simulink model "Simulation_Nonlinear_MRAC"  (R2023b)
settings: Solver=VariableStepAuto  StartTime=0.0  StopTime=Tsim  RelTol=1e-3
undefined symbols (not defined in the file): a, am, amplitude, b, BETA, BETA_m, bias, bm, epsilon, frequency, IC_P, IC_Pm, period, phase_delay, pulse_width, SAT_ACTIVE, SIGNAL_NR, Tsim, w, WEIGHT_UPDATE, wm
libraries: simulink x1
settings Model: Creator=dalimwahby  LastModifiedBy=dalimwahby

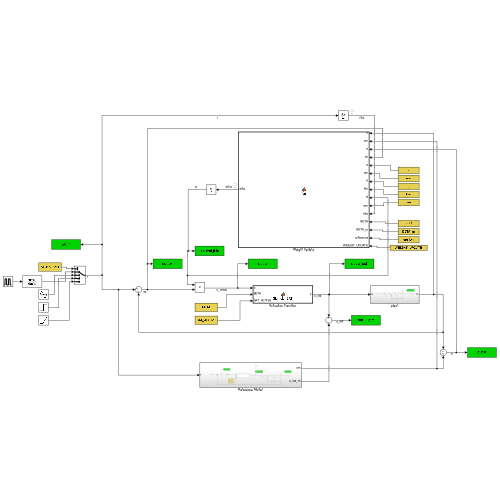
[thumbnail: Simulink's stored preview of the top-level diagram]
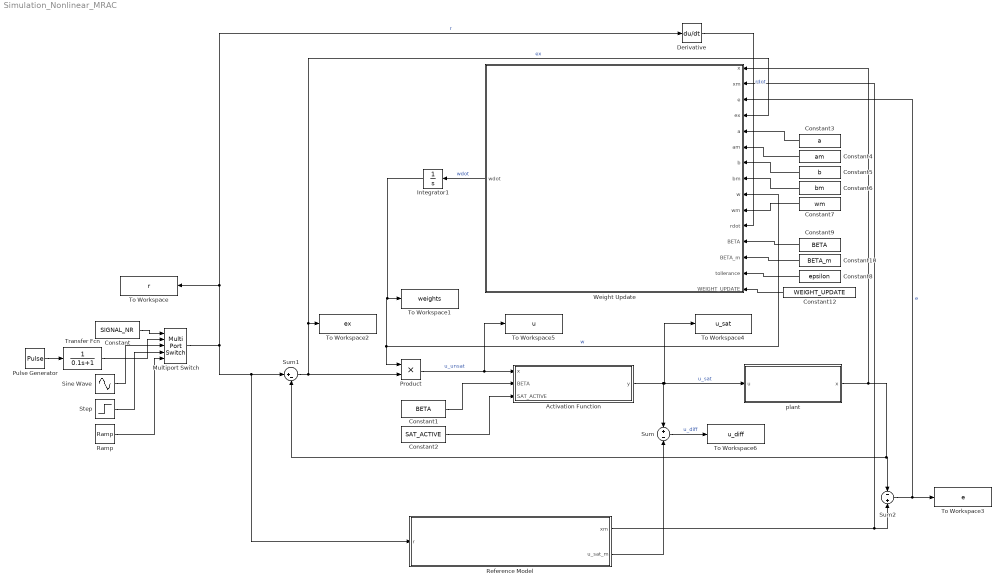
== system Simulation_Nonlinear_MRAC ==
  Activation Function : MATLAB Function  TreatAsAtomicUnit=on
  Constant : Constant  Value=SIGNAL_NR
  Constant1 : Constant  Value=BETA
  Constant10 : Constant  Value=BETA_m
  Constant12 : Constant  Value=WEIGHT_UPDATE
  Constant2 : Constant  Value=SAT_ACTIVE
  Constant3 : Constant  Value=a
  Constant4 : Constant  Value=am
  Constant5 : Constant  Value=b
  Constant6 : Constant  Value=bm
  Constant7 : Constant  Value=wm
  Constant8 : Constant  Value=epsilon
  Constant9 : Constant  Value=BETA
  Derivative : Derivative
  Integrator1 : Integrator  InitialCondition=w
  Multiport Switch : MultiPortSwitch  Inputs=4  SaturateOnIntegerOverflow=off  InputSameDT=off
  Product : Product
  Pulse Generator : DiscretePulseGenerator  PulseType=Time based  Amplitude=amplitude  Period=period  PulseWidth=pulse_width*100  PhaseDelay=phase_delay
  Ramp : simulink/Sources/Ramp  slope=1/Tsim  start=0  InitialOutput=0
  Reference Model : Subsystem
  Sine Wave : Sin  Amplitude=amplitude  Bias=bias  Frequency=frequency  SampleTime=0
  Step : Step  Time=phase_delay  After=amplitude  SampleTime=0
  Sum : Sum  Inputs=+-
  Sum1 : Sum  Inputs=|+-
  Sum2 : Sum  Inputs=-+
  To Workspace : ToWorkspace  VariableName=r  SaveFormat=Timeseries  SampleTime=-1
  To Workspace1 : ToWorkspace  VariableName=weights  SaveFormat=Timeseries  SampleTime=-1
  To Workspace2 : ToWorkspace  VariableName=ex  SaveFormat=Timeseries  SampleTime=-1
  To Workspace3 : ToWorkspace  VariableName=e  SaveFormat=Timeseries  SampleTime=-1
  To Workspace4 : ToWorkspace  VariableName=u_sat  SaveFormat=Timeseries  SampleTime=-1
  To Workspace5 : ToWorkspace  VariableName=u  SaveFormat=Timeseries  SampleTime=-1
  To Workspace6 : ToWorkspace  VariableName=u_diff  SaveFormat=Timeseries  SampleTime=-1
  Transfer Fcn : TransferFcn  Denominator=[0.1 1]
  Weight Update : MATLAB Function  TreatAsAtomicUnit=on
  plant : Subsystem
  wires:
  Multiport Switch/1 -> Sum1/1, Reference Model/1(r), Derivative/1, To Workspace/1  "r"
  Sine Wave/1 -> Multiport Switch/3
  Constant/1 -> Multiport Switch/1
  Step/1 -> Multiport Switch/4
  Reference Model/1(xm) -> Sum2/2, Weight Update/2(xm)
  Product/1 -> To Workspace5/1, Activation Function/1(x)  "u_unsat"
  Activation Function/1(y) -> plant/1(u), To Workspace4/1, Sum/1  "u_sat"
  Constant1/1 -> Activation Function/2(BETA)
  Constant2/1 -> Activation Function/3(SAT_ACTIVE)
  Sum1/1 -> To Workspace2/1, Weight Update/4(ex), Product/2  "ex"
  Sum2/1 -> Weight Update/3(e), To Workspace3/1  "e"
  Integrator1/1 -> To Workspace1/1, Weight Update/9(w), Product/1  "w"
  Weight Update/1(wdot) -> Integrator1/1  "wdot"
  plant/1(x) -> Weight Update/1(x), Sum2/1, Sum1/2
  Constant3/1 -> Weight Update/5(a)
  Constant4/1 -> Weight Update/6(am)
  Constant7/1 -> Weight Update/10(wm)
  Constant6/1 -> Weight Update/8(bm)
  Constant5/1 -> Weight Update/7(b)
  Derivative/1 -> Weight Update/11(rdot)  "rdot"
  Constant8/1 -> Weight Update/14(tollerance)
  Constant9/1 -> Weight Update/12(BETA)
  Constant10/1 -> Weight Update/13(BETA_m)
  Constant12/1 -> Weight Update/15(WEIGHT_UPDATE)
  Sum/1 -> To Workspace6/1  "u_diff"
  Reference Model/2(u_sat_m) -> Sum/2
  Ramp/1 -> Multiport Switch/5
  Pulse Generator/1 -> Transfer Fcn/1
  Transfer Fcn/1 -> Multiport Switch/2

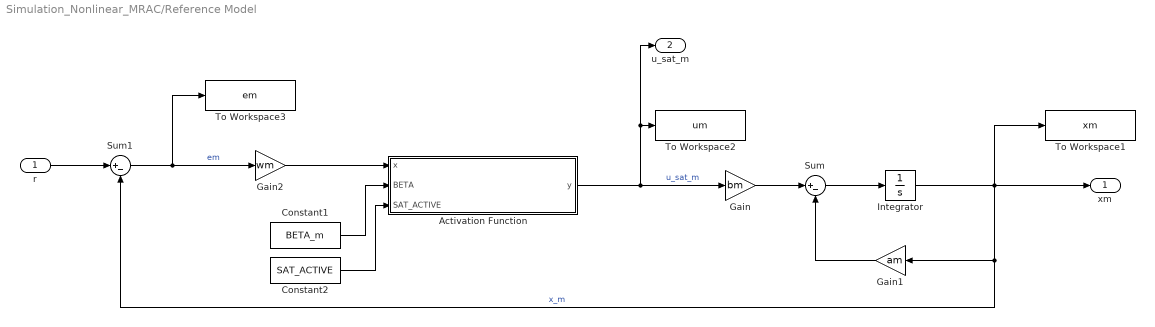
== system Simulation_Nonlinear_MRAC/Reference Model ==
  r : Inport
  Activation Function : MATLAB Function  TreatAsAtomicUnit=on
  Constant1 : Constant  Value=BETA_m
  Constant2 : Constant  Value=SAT_ACTIVE
  Gain : Gain  Gain=bm
  Gain1 : Gain  Gain=am
  Gain2 : Gain  Gain=wm
  Integrator : Integrator  InitialCondition=IC_Pm
  Sum : Sum  Inputs=|+-
  Sum1 : Sum  Inputs=|+-
  To Workspace1 : ToWorkspace  VariableName=xm  SaveFormat=Timeseries  SampleTime=-1
  To Workspace2 : ToWorkspace  VariableName=um  SaveFormat=Timeseries  SampleTime=-1
  To Workspace3 : ToWorkspace  VariableName=em  SaveFormat=Timeseries  SampleTime=-1
  xm : Outport
  u_sat_m : Outport  Port=2
  wires:
  Constant2/1 -> Activation Function/3(SAT_ACTIVE)
  Sum/1 -> Integrator/1
  Constant1/1 -> Activation Function/2(BETA)
  Gain1/1 -> Sum/2
  Activation Function/1(y) -> u_sat_m/1, To Workspace2/1, Gain/1  "u_sat_m"
  Integrator/1 -> Sum1/2, Gain1/1, xm/1, To Workspace1/1  "x_m"
  Gain/1 -> Sum/1
  Gain2/1 -> Activation Function/1(x)
  r/1 -> Sum1/1
  Sum1/1 -> To Workspace3/1, Gain2/1  "em"

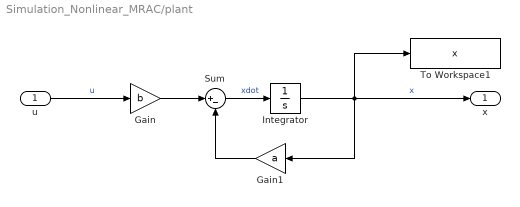
== system Simulation_Nonlinear_MRAC/plant ==
  u : Inport
  Gain : Gain  Gain=b
  Gain1 : Gain  Gain=a
  Integrator : Integrator  InitialCondition=IC_P
  Sum : Sum  Inputs=|+-
  To Workspace1 : ToWorkspace  VariableName=x  SaveFormat=Timeseries  SampleTime=-1
  x : Outport
  wires:
  u/1 -> Gain/1  "u"
  Sum/1 -> Integrator/1  "xdot"
  Integrator/1 -> Gain1/1, x/1, To Workspace1/1  "x"
  Gain1/1 -> Sum/2
  Gain/1 -> Sum/1

== matlab function Simulation_Nonlinear_MRAC/Activation Function ==
  data: x input; y output; BETA input; SAT_ACTIVE input
function y = Sigmoid_SAT(x, BETA, SAT_ACTIVE)
    if SAT_ACTIVE==1
        y = (2*(1-exp(-BETA.*x)))./(BETA*(1+exp(-BETA.*x)));
    else
        y = x;
    end
end

== matlab function Simulation_Nonlinear_MRAC/Reference Model/Activation Function ==
  data: x input; y output; BETA input; SAT_ACTIVE input
function y = Sigmoid_SAT(x, BETA, SAT_ACTIVE)
    if SAT_ACTIVE==1
        y = (2*(1-exp(-BETA.*x)))./(BETA*(1+exp(-BETA.*x)));
    else
        y = x;
    end
end

== matlab function Simulation_Nonlinear_MRAC/Weight Update ==
  data: x input; xm input; e input; wdot output; ex input; a input; am input; b input; bm input; w input; wm input; rdot input; BETA input; BETA_m input; tollerance input; WEIGHT_UPDATE input
function wdot = fcn(x, xm, e, ex, a, am, b ,bm, w, wm, rdot, BETA, BETA_m, tollerance, WEIGHT_UPDATE)
if WEIGHT_UPDATE==1
    %% If ex is equal to zero, do not update the weights due to zero division
    if abs(ex)<=tollerance
        wdot=0;

    else
        %% System
        input_ex = w*ex;
        sigma_ex = (2*(1-exp(-BETA.*input_ex)))./(BETA*(1+exp(-BETA.*input_ex)));
        
        xdot = -a*x+b*sigma_ex;
        
        exdot = rdot-xdot;
    
        dsigma_ex = (4*exp(-BETA.*input_ex))./((1+exp(-BETA.*input_ex)).^2);
        
        %% Model reference
        input_em = wm*ex;
        %sigma_em = (2*(1-exp(-BETA_m.*input_em)))./(BETA_m*(1+exp(-BETA_m.*input_em)));

        %xmdot = -am*xm+bm*sigma_em;
        
        %emdot = rdot-xmdot;
        emdot=exdot;
    
        dsigma_em = (4*exp(-BETA_m.*input_em))./((1+exp(-BETA_m.*input_em)).^2);
    
    
        %% Time derivative of weights
        wdot = ((1/(ex*b*dsigma_ex))*(e + (a-am)*xdot + bm*dsigma_em*wm*emdot)-((w/ex)*exdot));

    end
else
    wdot=0;
end
